simulink model "Lab_9"  (R2023a)
settings: Solver=VariableStepAuto  StartTime=0.0  StopTime=10.0  RelTol=1e-3
libraries: spsSawtoothGeneratorLib x1
settings Model: Creator=mluser  LastModifiedBy=mluser

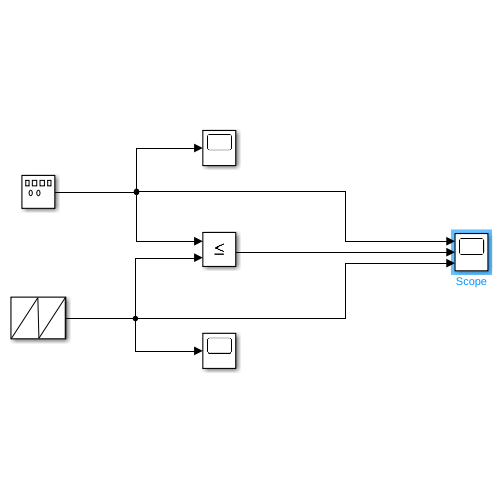
[thumbnail: Simulink's stored preview of the top-level diagram]
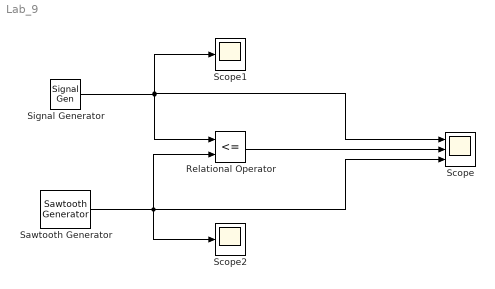
== system Lab_9 ==
  Relational Operator : RelationalOperator  Operator=<=  OutDataTypeStr=boolean  RndMeth=Simplest  InputSameDT=off
  Sawtooth Generator : spsSawtoothGeneratorLib/Sawtooth Generator  Freq=1  Phase=0  Ts=0
  Scope : Scope  NumInputPorts=3
  Scope1 : Scope
  Scope2 : Scope
  Signal Generator : SignalGenerator  Frequency=0.5  Units=rad/sec
  wires:
  Sawtooth Generator/1 -> Scope2/1, Scope/3, Relational Operator/2
  Signal Generator/1 -> Relational Operator/1, Scope1/1, Scope/1
  Relational Operator/1 -> Scope/2
